simulink model "POSH_Test"  (R2016a)
settings: Solver=FixedStepDiscrete  StartTime=0.0  StopTime=16  FixedStep=0.005  RelTol=1e-3
undefined symbols (not defined in the file): sigbuilder_block
libraries: POSH x1
settings Model: Creator=oelkawok  LastModifiedBy=oelkawok
settings DataIOCC: SaveOutput=off  SaveTime=off

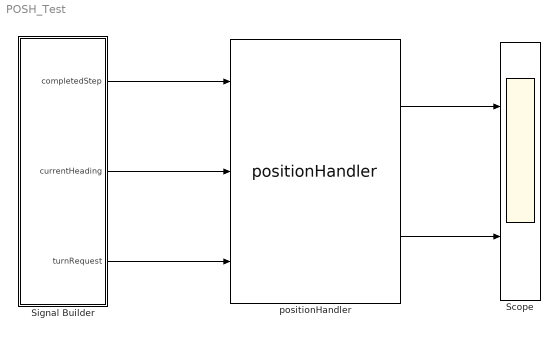
== system POSH_Test ==
  Scope : Scope  NumInputPorts=2
  Signal Builder : Subsystem  Tag=STV Subsys  LoadFcn=sigbuilder_block('load',[-679.8 87.6 550.8 400.2 ]);  StartFcn=sigbuilder_block('start');  StopFcn=sigbuilder_block('stop');  ClipboardFcn=sigbuilder_block('clipboard');  mask(Sigbuilder block){}
      mask help: Simulink:masks:SigbuilderBlock_MD
      mask init:
      | if ~strcmp(get_param(bdroot(gcbh),'SimulationStatus'),'stopped') tuvar = sigbuilder_block('maskInit'); end
      settings: CopyFcn=sigbuilder_block('copy');  DeleteFcn=sigbuilder_block('delete');  ModelCloseFcn=sigbuilder_block('modelClose');  PreSaveFcn=sigbuilder_block('preSave');  PauseFcn=sigbuilder_block('pause');  ContinueFcn=sigbuilder_block('continue');  NameChangeFcn=sigbuilder_block('namechange');  OpenFcn=sigbuilder_block('open',[437.6 199.2 550.4 400 ]);  CloseFcn=sigbuilder_block('close');
      mask Display: plot(0, 0, 100, 100,[2, 2, 32, 32, 2], [68, 8, 8, 68, 68],[32, 2], [38, 38], [32, 19, 2],[53, 60, 44], [32, 17, 17, 2],[16, 16, 31, 31]);txt = getActiveGroup(gcbh);text(2, 100, txt,'verticalAlignment', 'top');
  positionHandler : POSH/positionHandler
  wires:
  Signal Builder/1(completedStep) -> positionHandler/1
  Signal Builder/2(currentHeading) -> positionHandler/2
  Signal Builder/3(turnRequest) -> positionHandler/3
  positionHandler/1 -> Scope/1
  positionHandler/2 -> Scope/2

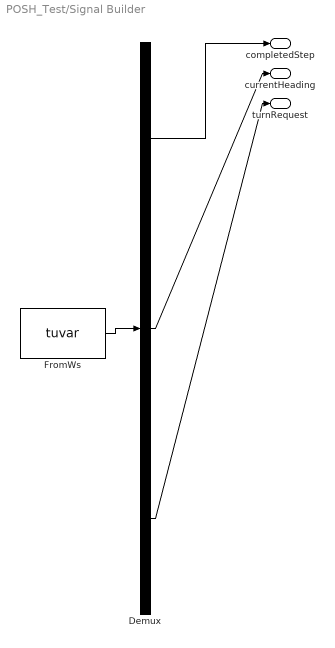
== system POSH_Test/Signal Builder ==
  Demux : Demux  Tag=STV Demux  Outputs=3
  FromWs : FromWorkspace  Tag=STV FromWs  VariableName=tuvar  SampleTime=0
      SigBuilderData=|
      | common.afterFinalStr = 'Extrapolate'
      | common.sampleTime = 0
      | dataSet.timeRange = [0 10]
      | dataSet.name = 'Group 1'
      | sbobj.Groups.Name = 'Group 1'
      | sbobj.Groups.Signals(1).Name = 'completedStep'
      | sbobj.Groups.Signals(1).XData = [0 1.8 1.8 2.16 2.16 3.66 3.66 3.8 3.8 5.42 5.42 5.64 5.64 7.84 7.84 7.9 7.9 10]
      | sbobj.Groups.Signals(1).YData = [0 0 1 1 0 0 1 1 0 0 1 1 0 0 1 1 0 0]
      | sbobj.Groups.Signals(2).Name = 'currentHeading'
      | sbobj.Groups.Signals(2).XData = [0 0.26 0.26 2.5 2.5 2.9 2.9 4.54 4.54 4.84 4.84 6.38 6.38 6.88 6.88 10]
      | sbobj.Groups.Signals(2).YData = [400 400 180 180 400 400 90 90 400 400 0 0 400 400 270 270]
      | sbobj.Groups.Signals(3).Name = 'turnRequest'
      | sbobj.Groups.Signals(3).XData = [0 0.18 0.18 2.44 2.44 6.26 6.26 10]
      | sbobj.Groups.Signals(3).YData = [0 0 1 1 2 2 1 1]
  completedStep : Outport  Tag=STV Outport
  currentHeading : Outport  Tag=STV Outport  Port=2
  turnRequest : Outport  Tag=STV Outport  Port=3
  wires:
  Demux/1 -> completedStep/1
  FromWs/1 -> Demux/1
  Demux/2 -> currentHeading/1
  Demux/3 -> turnRequest/1
